simulink model "TEG"  (R2024a)
settings: Solver=VariableStepAuto  StartTime=0.0  StopTime=5.6  RelTol=1e-3
undefined symbols (not defined in the file): delta_T, m, RL, Vm, Wm
settings Model: Creator=charles  LastModifiedBy=mdnau
settings SolverCC: AlgebraicLoopSolver=TrustRegion
settings DebuggingCC: UnconnectedInputMsg=warning  UnconnectedOutputMsg=warning  UnconnectedLineMsg=warning
settings ModelReferenceCC: EnableRefExpFcnMdlSchedulingChecks=on
settings SFSimCC: CustomCodeUndefinedFunction=UseInterfaceOnly
settings RTWCC: GPUComputeCapability=3.5

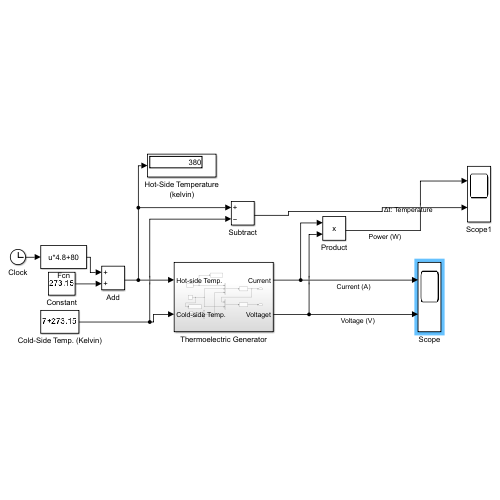
[thumbnail: Simulink's stored preview of the top-level diagram]
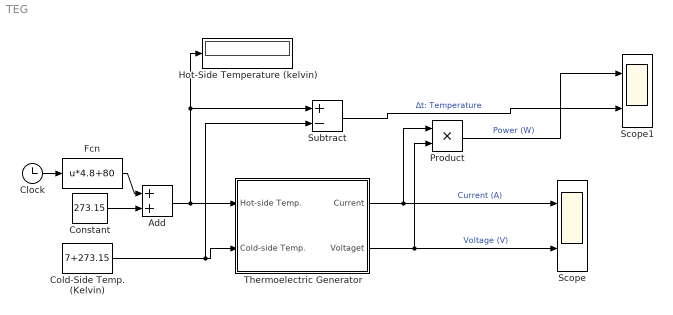
== system TEG ==
  Add : Sum
  Clock : Clock
  Cold-Side Temp. (Kelvin) : Constant  Value=7+273.15
  Constant : Constant  Value=273.15
  Fcn : Fcn  Expr=u*4.8+80
  Hot-Side Temperature (kelvin) : Display
  Product : Product
  Scope : Scope  NumInputPorts=2
  Scope1 : Scope  NumInputPorts=2
  Subtract : Sum  Inputs=+-
  Thermoelectric Generator : Subsystem
  wires:
  Cold-Side Temp. (Kelvin)/1 -> Subtract/2, Thermoelectric Generator/2(Cold-side Temp.)
  Add/1 -> Subtract/1, Hot-Side Temperature (kelvin)/1, Thermoelectric Generator/1(Hot-side Temp.)
  Thermoelectric Generator/2(Voltaget) -> Product/2, Scope/2  "Voltage (V)"
  Thermoelectric Generator/1(Current) -> Product/1, Scope/1  "Current (A)"
  Product/1 -> Scope1/1  "Power (W)"
  Clock/1 -> Fcn/1
  Constant/1 -> Add/2
  Subtract/1 -> Scope1/2  "Δt: Temperature"
  Fcn/1 -> Add/1

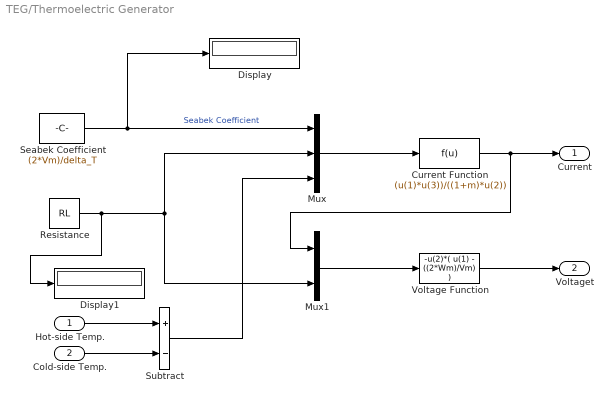
== system TEG/Thermoelectric Generator ==
  Hot-side Temp. : Inport
  Cold-side Temp. : Inport  Port=2
  Current Function : Fcn  Expr=(u(1)*u(3))/((1+m)*u(2))
  Display : Display
  Display1 : Display
  Mux : Mux  Inputs=3
  Mux1 : Mux  Inputs=2
  Resistance : Constant  Value=RL
  Seabek Coefficient : Constant  Value=(2*Vm)/delta_T
  Subtract : Sum  Inputs=+-
  Voltage Function : Fcn  Expr=-u(2)*( u(1) - ((2*Wm)/Vm) )
  Current : Outport  VectorParamsAs1DForOutWhenUnconnected=off
  Voltaget : Outport  Port=2  VectorParamsAs1DForOutWhenUnconnected=off
  wires:
  Hot-side Temp./1 -> Subtract/1
  Cold-side Temp./1 -> Subtract/2
  Current Function/1 -> Current/1, Mux1/1
  Mux1/1 -> Voltage Function/1
  Resistance/1 -> Display1/1, Mux1/2, Mux/2
  Seabek Coefficient/1 -> Display/1, Mux/1  "Seabek Coefficient"
  Voltage Function/1 -> Voltaget/1
  Subtract/1 -> Mux/3
  Mux/1 -> Current Function/1
